simulink model "chap6_8sim"  (R2016b)
settings: Solver=ode45  StartTime=0.0  StopTime=10.0  RelTol=1e-3
settings Model: Creator=guoshaopan  LastModifiedBy=guoshaopan

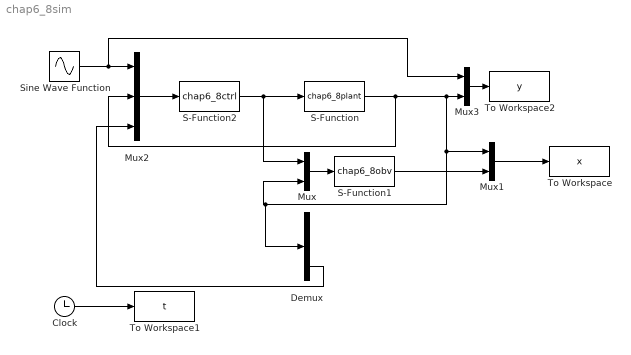
== system chap6_8sim ==
  Clock : Clock
  Demux : Demux  Outputs=3
  Mux : Mux  Inputs=2
  Mux1 : Mux  Inputs=2
  Mux2 : Mux  Inputs=3
  Mux3 : Mux  Inputs=2
  S-Function : S-Function  FunctionName=chap6_8plant  SFunctionDeploymentMode=off  EnableBusSupport=off
  S-Function1 : S-Function  FunctionName=chap6_8obv  SFunctionDeploymentMode=off  EnableBusSupport=off
  S-Function2 : S-Function  FunctionName=chap6_8ctrl  SFunctionDeploymentMode=off  EnableBusSupport=off
  Sine Wave Function : Sin  SampleTime=0
  To Workspace : ToWorkspace  VariableName=x  SampleTime=-1
  To Workspace1 : ToWorkspace  VariableName=t  SampleTime=-1
  To Workspace2 : ToWorkspace  VariableName=y  SampleTime=-1
  wires:
  Mux1/1 -> To Workspace/1
  Clock/1 -> To Workspace1/1
  Sine Wave Function/1 -> Mux3/1, Mux2/1
  Mux2/1 -> S-Function2/1
  S-Function2/1 -> Mux/1, S-Function/1
  Mux3/1 -> To Workspace2/1
  S-Function/1 -> Mux2/2, Mux1/1, Demux/1, Mux/2, Mux3/2
  Mux/1 -> S-Function1/1
  S-Function1/1 -> Mux1/2
  Demux/3 -> Mux2/3
